simulink model "BWQWFPIDbzls"  (Simulink 5.0)
settings: Solver=ode4  StartTime=0.0  StopTime=1000  FixedStep=20  RelTol=1e-3
settings Model: LastModifiedBy=ThinkPad  RTWOptions="-aEnforceIntegerDowncast=1 -aExtMode=0 -aExtModeTesting=0 -aFoldNonRolledExpr=1 -aForceParamTrailComments=0 -aGenerateComments=1 -aGenerateReport=0 -aIgnoreCustomStorageClasses=1 -aIncDataTypeInIds=0 -aIncHierarchyInIds=0 -aInlineInvariantSignals=0 -aInlinedPrmAccess=\"Literals\" -aLocalBlockOutputs=1 -aLogVarNameModifier=\"rt_\" -aMaxRTWIdLen=31 -aPrefixModelToSubsysFcnNames=1 -aRTWVerbose=1 -aRollThreshold=5 -aShowEliminatedStatements=0"

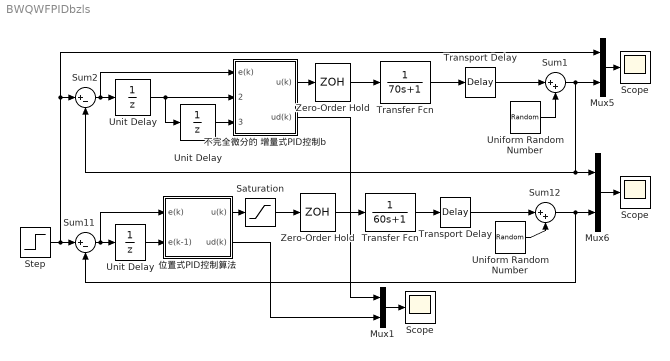
== system BWQWFPIDbzls ==
  " Scope " : Scope
      settings: YMin=-0.2  YMax=1.2  MaxDataPoints=500000
  " Unit Delay " : UnitDelay  SampleTime=20
  Mux1 : Mux  Inputs=2
  Mux5 : Mux  Inputs=2
  Mux6 : Mux  Inputs=2
  "Saturation " : Saturate  UpperLimit=10  LowerLimit=-10
  Scope : Scope
      settings: YMin=-0.2  YMax=1.2  SaveName=ScopeData2  MaxDataPoints=500000
  "Scope " : Scope
      settings: YMin=-3.5  YMax=1  SaveName=ScopeData3  MaxDataPoints=500000
  Step : Step  Time=0  SampleTime=20
  Sum1 : Sum  Inputs=|++  SaturateOnIntegerOverflow=on
  Sum11 : Sum  Inputs=|+-  SaturateOnIntegerOverflow=on
  Sum12 : Sum  Inputs=|++  SaturateOnIntegerOverflow=on
  Sum2 : Sum  Inputs=|+-  SaturateOnIntegerOverflow=on
  Transfer Fcn : TransferFcn  Denominator=[70 1]
  "Transfer Fcn " : TransferFcn  Denominator=[60 1]
  Transport Delay : TransportDelay  DelayTime=80
  "Transport Delay " : TransportDelay  DelayTime=80
  Uniform Random Number : UniformRandomNumber  Minimum=-0.01  Maximum=0.01  SampleTime=20
  "Uniform Random Number " : UniformRandomNumber  Minimum=-0.01  Maximum=0.01  SampleTime=0
  Unit Delay : UnitDelay  SampleTime=20
  "Unit Delay " : UnitDelay  SampleTime=20
  Zero-Order Hold : ZeroOrderHold  SampleTime=20
  "Zero-Order Hold " : ZeroOrderHold  SampleTime=20
  不完全微分的 增量式PID控制b : Subsystem
  "位置式PID控制算法 " : Subsystem
  wires:
  Step/1 -> Sum11/1, Sum2/1, Mux5/1
  "Transfer Fcn "/1 -> "Transport Delay "/1
  "位置式PID控制算法 "/1(u(k)) -> "Saturation "/1
  "Unit Delay "/1 -> "位置式PID控制算法 "/2(e(k-1))
  Sum11/1 -> "Unit Delay "/1, "位置式PID控制算法 "/1(e(k))
  "Zero-Order Hold "/1 -> "Transfer Fcn "/1
  "Uniform Random Number "/1 -> Sum12/2
  "Transport Delay "/1 -> Sum12/1
  Mux6/1 -> Scope/1
  Sum12/1 -> Sum11/2, Mux6/2
  "Saturation "/1 -> "Zero-Order Hold "/1
  Transfer Fcn/1 -> Transport Delay/1
  不完全微分的 增量式PID控制b/1(u(k)) -> Zero-Order Hold/1
  Sum2/1 -> Unit Delay/1, 不完全微分的 增量式PID控制b/1(e(k))
  Mux5/1 -> "Scope "/1
  Uniform Random Number/1 -> Sum1/2
  Transport Delay/1 -> Sum1/1
  Sum1/1 -> Sum2/2, Mux6/1, Mux5/2
  Zero-Order Hold/1 -> Transfer Fcn/1
  " Unit Delay "/1 -> 不完全微分的 增量式PID控制b/3(e(k-2))
  Unit Delay/1 -> 不完全微分的 增量式PID控制b/2(e(k-1)), " Unit Delay "/1
  Mux1/1 -> " Scope "/1
  不完全微分的 增量式PID控制b/2(ud(k)) -> Mux1/1
  "位置式PID控制算法 "/2(ud(k)) -> Mux1/2

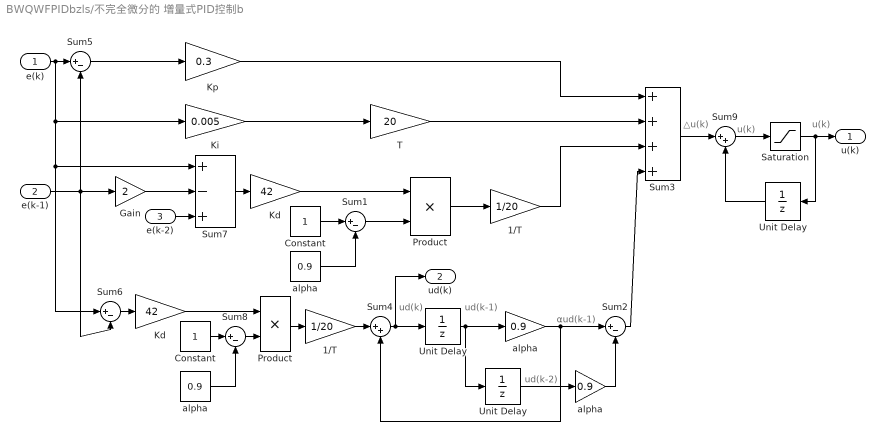
== system BWQWFPIDbzls/不完全微分的 增量式PID控制b ==
  note: △u(k)
  note: u(k)
  note: u(k)
  note: ud(k)
  note: ud(k-1)
  note: ud(k-2)
  note: αud(k-1)
  e(k) : Inport
  e(k-1) : Inport  Port=2
  e(k-2) : Inport  Port=3
  " Product  " : Product  SaturateOnIntegerOverflow=on
  " Saturation " : Saturate  UpperLimit=10  LowerLimit=-10
  " Unit Delay" : UnitDelay  SampleTime=20
  " Unit Delay " : UnitDelay  SampleTime=20
  " alpha" : Gain  Gain=0.9  SaturateOnIntegerOverflow=on
  " alpha " : Gain  Gain=0.9  SaturateOnIntegerOverflow=on
  1/T : Gain  Gain=1/20  SaturateOnIntegerOverflow=on
  "1/T " : Gain  Gain=1/20  SaturateOnIntegerOverflow=on
  Constant : Constant
  "Constant " : Constant
  Gain : Gain  Gain=2  SaturateOnIntegerOverflow=on
  Kd : Gain  Gain=42  SaturateOnIntegerOverflow=on
  "Kd " : Gain  Gain=42  SaturateOnIntegerOverflow=on
  Ki : Gain  Gain=0.005  SaturateOnIntegerOverflow=on
  Kp : Gain  Gain=0.3  SaturateOnIntegerOverflow=on
  "Product " : Product  SaturateOnIntegerOverflow=on
  Sum{1..2,5..6,8} (5 alike) : Sum  Inputs=|+-  SaturateOnIntegerOverflow=on
  Sum3 : Sum  Inputs=++++  SaturateOnIntegerOverflow=on
  Sum4 : Sum  Inputs=|++  SaturateOnIntegerOverflow=on
  Sum7 : Sum  Inputs=+-+  SaturateOnIntegerOverflow=on
  Sum9 : Sum  Inputs=|++  SaturateOnIntegerOverflow=on
  T : Gain  Gain=20  SaturateOnIntegerOverflow=on
  Unit Delay : UnitDelay  Orientation=left  SampleTime=20
  alpha : Constant  Value=0.9
  "alpha " : Constant  Value=0.9
  u(k) : Outport
  ud(k) : Outport  Port=2
  wires:
  Sum5/1 -> Kp/1
  e(k-1)/1 -> Sum5/2, Gain/1, Sum6/2
  e(k)/1 -> Sum5/1, Ki/1, Sum7/1, Sum6/1
  Ki/1 -> T/1
  Gain/1 -> Sum7/2
  e(k-2)/1 -> Sum7/3
  Sum7/1 -> Kd/1
  T/1 -> Sum3/2
  Kp/1 -> Sum3/1
  Sum3/1 -> Sum9/1
  Sum9/1 -> " Saturation "/1
  " Saturation "/1 -> Unit Delay/1, u(k)/1
  Unit Delay/1 -> Sum9/2
  Constant/1 -> Sum1/1
  alpha/1 -> Sum1/2
  Sum1/1 -> " Product  "/2
  " Product  "/1 -> 1/T/1
  1/T/1 -> Sum3/3
  Kd/1 -> " Product  "/1
  " Unit Delay "/1 -> " Unit Delay"/1, " alpha"/1
  " alpha"/1 -> Sum2/1, Sum4/2
  " Unit Delay"/1 -> " alpha "/1
  " alpha "/1 -> Sum2/2
  "Constant "/1 -> Sum8/1
  "alpha "/1 -> Sum8/2
  Sum8/1 -> "Product "/2
  "Kd "/1 -> "Product "/1
  Sum6/1 -> "Kd "/1
  "Product "/1 -> "1/T "/1
  Sum2/1 -> Sum3/4
  "1/T "/1 -> Sum4/1
  Sum4/1 -> " Unit Delay "/1, ud(k)/1

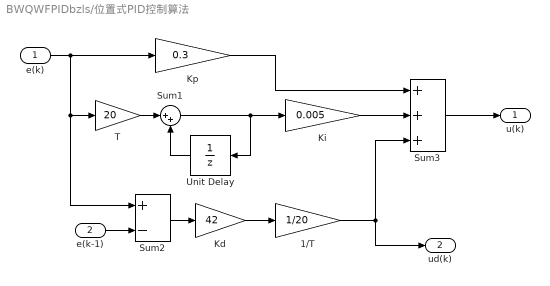
== system BWQWFPIDbzls/位置式PID控制算法  ==
  e(k) : Inport
  e(k-1) : Inport  Port=2
  1/T : Gain  Gain=1/20  SaturateOnIntegerOverflow=on
  Kd : Gain  Gain=42  SaturateOnIntegerOverflow=on
  Ki : Gain  Gain=0.005  SaturateOnIntegerOverflow=on
  Kp : Gain  Gain=0.3  SaturateOnIntegerOverflow=on
  Sum1 : Sum  Inputs=|++  SaturateOnIntegerOverflow=on
  Sum2 : Sum  Inputs=+-  SaturateOnIntegerOverflow=on
  Sum3 : Sum  Inputs=+++  SaturateOnIntegerOverflow=on
  T : Gain  Gain=20  SaturateOnIntegerOverflow=on
  "Unit Delay " : UnitDelay  Orientation=left  SampleTime=20
  u(k) : Outport
  ud(k) : Outport  Port=2
  wires:
  Sum2/1 -> Kd/1
  e(k)/1 -> Kp/1, Sum2/1, T/1
  Kp/1 -> Sum3/1
  Ki/1 -> Sum3/2
  Sum3/1 -> u(k)/1
  Kd/1 -> 1/T/1
  e(k-1)/1 -> Sum2/2
  1/T/1 -> Sum3/3, ud(k)/1
  Sum1/1 -> "Unit Delay "/1, Ki/1
  "Unit Delay "/1 -> Sum1/2
  T/1 -> Sum1/1
